simulink library "RobotStateLibrary_R2020b"  (R2020b)
settings: Solver=VariableStepAuto  StartTime=0.0  StopTime=10.0  RelTol=1e-3
undefined symbols (not defined in the file or in its folder): Aeq_add, baseFrameName1, basePosePortName, beq_add, config, Config, ConfigRobot1, configSafety, contactFrame1Name, contactFrame2Name, frame1, frame2, frame3, frame4, frameName2, gainStruct, RegStruct, regularization, sampleTime, tollerance, useConstraint, weight
libraries: WBToolboxLibrary x38, $bdroot x32
(part 1 of 2)
settings Model: Creator=lorenzorapetti  LastModifiedBy=lorenzorapetti

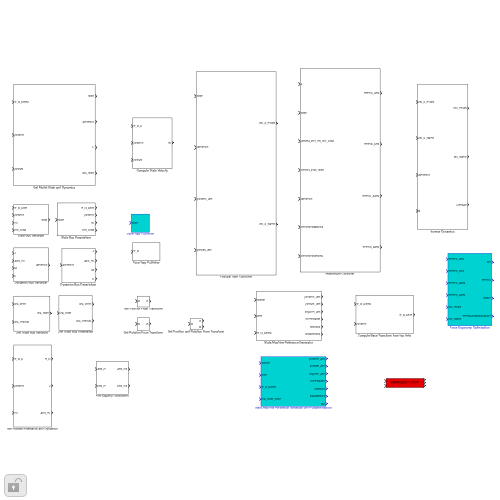
[thumbnail: Simulink's stored preview of the top-level diagram]
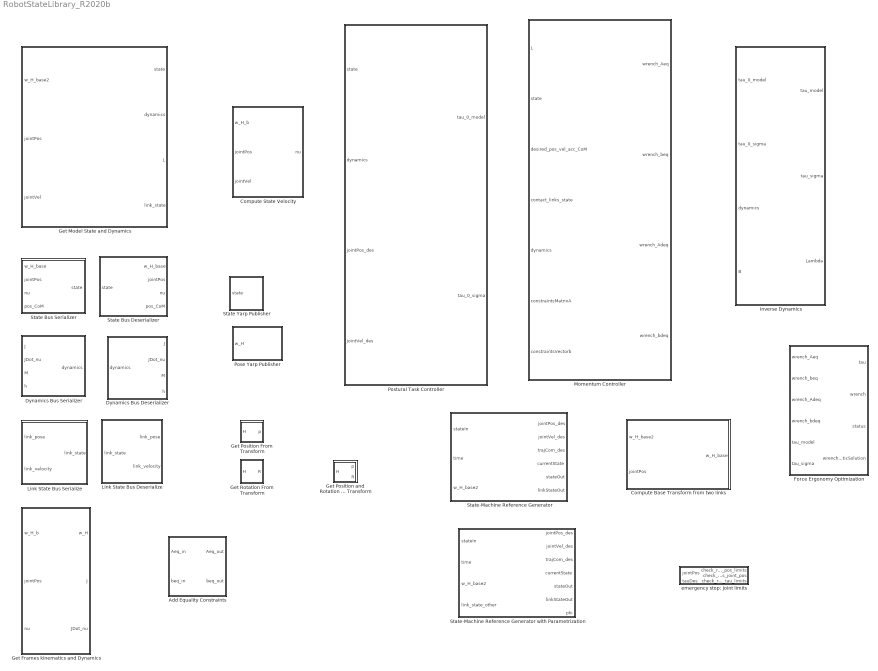
== system RobotStateLibrary_R2020b ==
  Add Equality Constraints : Subsystem  mask{Aeq_add=Aeq_add, beq_add=beq_add}
      mask prompts: Aeq_add "Additional Constraints A"; beq_add "Additional Constraints b"
  Compute Base Transform from two links : Subsystem  mask{frameName1=baseFrameName1, frameName2=frameName2}
      mask prompts: frameName1 "Frame name 1"; frameName2 "Frame name 2"
      mask TypeOptions frameName1: Relative transform base2_H_base/frameName
      mask TypeOptions frameName2: Relative transform base2_H_base1/frameName
  Compute State Velocity : Subsystem  mask{frameName1=contactFrame1Name, frameName2=contactFrame2Name, regularization=regularization}
      mask prompts: frameName1 "Contact Frame 1"; frameName2 "Contact Frame 2"
      mask TypeOptions frameName1: Contacts Jacobians/Jacobian Contact 1/frameName
      mask TypeOptions frameName2: Contacts Jacobians/Jacobian Contact 2/frameName
  Dynamics Bus Deserializer : Subsystem
  Dynamics Bus Serializer : Subsystem
  Force Ergonomy Optimization : Subsystem  mask{InvTol=tollerance, regularizationHessian=regularization, minimizationWeight=weight}
      mask prompts: InvTol "Pseudoinverse Tollerance"; regularizationHessian "Regularization Hessian"; minimizationWeight "Minimization Weight"
  Get Frames kinematics and Dynamics : Subsystem  mask{frame1=frame1, frame2=frame2, frame3=frame3, frame4=frame4, nDoF=1}
      mask prompts: frame1 "Frame 1"; frame2 "Frame 2"; frame3 "Frame 3"; frame4 "Frame 4"; nDoF "Model DoF"
      mask TypeOptions nDoF:
      | CoM6D ->
      | CoMXYZ3/OutputSizes
  Get Model State and Dynamics : Subsystem  mask{nDoF=1, regularization=0, contactFrame1Name=[], contactFrame2Name=[], frame1=[], frame2=[], frame3=[], frame4=[]}
      mask prompts: nDoF "Model DoF"; regularization "Base Velocity Regularization"; contactFrame1Name "Contact Frame 1"; contactFrame2Name "Contact Frame 2"; frame1 "Frame 1"; frame2 "Frame 2"; frame3 "Frame 3"; frame4 "Frame 4"
      mask TypeOptions nDoF: Get Frames kinematics and Dynamics/nDoF | Get Model Kinematics and Dynamics/nDoF
      mask TypeOptions regularization: Compute State Velocity/regularization
      mask TypeOptions contactFrame1Name: Compute State Velocity/frameName1
      mask TypeOptions contactFrame2Name: Compute State Velocity/frameName2
      mask TypeOptions frame1: Get Frames kinematics and Dynamics/frame1
      mask TypeOptions frame2: Get Frames kinematics and Dynamics/frame2
      mask TypeOptions frame3: Get Frames kinematics and Dynamics/frame3
      mask TypeOptions frame4: Get Frames kinematics and Dynamics/frame4
      mask DialogControl Container4 Prompt: Base Velocity Parameters
      mask DialogControl Container3 Prompt: Contact Frames
      mask DialogControl Container5 Prompt: Frames
  Get Position From Transform : Subsystem
  Get Position and Rotation From Transform : Subsystem
  Get Rotation From Transform : Subsystem
  Inverse Dynamics : Subsystem  mask{Reg=RegStruct, fixedLinkVelcityComponents=0}
      mask prompts: Reg "Regularization Values"; fixedLinkVelcityComponents "Fixed Link Velocity Components"
  Link State Bus Deserialize : Subsystem
  Link State Bus Serialize : Subsystem
  Momentum Controller : Subsystem  mask{GainMomentum=gainStruct, linksUseConstraintMatrix=useConstraint}
      mask prompts: GainMomentum "Momentum Control Gain"; linksUseConstraintMatrix "Use Force Constraint on Links"
  Pose Yarp Publisher : Subsystem  mask{portName=basePosePortName}
      mask prompts: portName "Pose Port Name"
      mask TypeOptions portName: base pose/portName
  Postural Task Controller : Subsystem  mask{GainPostural=gainStruct}
      mask prompts: GainPostural "Postural Task Gain"
  State Bus Deserializer : Subsystem
  State Bus Serializer : Subsystem
  State Yarp Publisher : Subsystem  mask{basePosePortName='/portname', jointPosPortName='/portname', nuPortName='/portname', posCoMPortName='/portname'}
      mask prompts: basePosePortName "Base Pose Port Name"; jointPosPortName "Joint Position Port Name"; nuPortName "State Velocity Port Name"; posCoMPortName "CoM Position Port Name"
      mask TypeOptions basePosePortName: Pose Yarp Publisher/portName
      mask TypeOptions jointPosPortName: joint position/portName
      mask TypeOptions nuPortName: nu/portName
      mask TypeOptions posCoMPortName: CoM position/portName
  State-Machine Reference Generator : Subsystem  mask{configStateMachine=config, sampleTime=sampleTime, frameName1=baseFrameName1, frameName2=baseFrameName1, regularization=regularization, nDoF=1, frame1=frame1, frame2=frame2, frame3=frame3, frame4=frame4}
      mask prompts: configStateMachine "State Machine Configuration"; sampleTime "Sample Time"; frameName1 "Contact Frame 1"; frameName2 "Contact Frame 2"; regularization "Base Veocity Regularization"; nDoF "Model DoF"; frame1 "Frame 1"; frame2 "Frame 2"; frame3 "Frame 3"; frame4 "Frame 4"
      mask TypeOptions sampleTime: MinimumJerkTrajectoryGenerator1/sampleTime | MinimumJerkTrajectoryGenerator2/sampleTime
      mask TypeOptions frameName1: Compute Base Transform from two links/frameName1 | Compute State Velocity/frameName1
      mask TypeOptions frameName2: Compute Base Transform from two links/frameName2 | Compute State Velocity/frameName2
      mask TypeOptions regularization: Compute State Velocity/regularization
      mask TypeOptions nDoF: Get Frames kinematics and Dynamics/nDoF
      mask TypeOptions frame1: Get Frames kinematics and Dynamics/frame1
      mask TypeOptions frame2: Get Frames kinematics and Dynamics/frame2
      mask TypeOptions frame3: Get Frames kinematics and Dynamics/frame3
      mask TypeOptions frame4: Get Frames kinematics and Dynamics/frame4
      mask DialogControl Container3 Prompt: Frames
  State-Machine Reference Generator with Parametrization : Subsystem  mask{configStateMachine=config, frameName1=frame1, frameName2=frame2, regularization=regularization, nDoF=ROBOT_DOF, frame1=frame1, frame2=frame2, frame3=frame3, frame4=frame4, settlingTime=1, sampleTime=1}
      mask prompts: configStateMachine "State Machine Configuration"; frameName1 "Contact Frame 1"; frameName2 "Contact Frame 2"; regularization "Base Veocity Regularization"; nDoF "Model DoF"; frame1 "Frame 1"; frame2 "Frame 2"; frame3 "Frame 3"; frame4 "Frame 4"; settlingTime "Settling Time"; sampleTime "Sample Time"
      mask TypeOptions frameName1: Compute Output State/frameName1 | Compute CoM Trajectory/frameName1
      mask TypeOptions frameName2: Compute Output State/frameName2 | Compute CoM Trajectory/frameName2
      mask TypeOptions regularization: Compute Output State/regularization
      mask TypeOptions nDoF: Compute Output State/nDoF
      mask TypeOptions frame1: Compute Output State/frame1
      mask TypeOptions frame2: Compute Output State/frame2
      mask TypeOptions frame3: Compute Output State/frame3
      mask TypeOptions frame4: Compute Output State/frame4
      mask TypeOptions settlingTime: Compute CoM Trajectory/settlingTime | Compute Output State/settlingTime
      mask TypeOptions sampleTime: Compute CoM Trajectory/sampleTime | Compute Output State/sampleTime
      mask DialogControl Container3 Prompt: Frames
      mask DialogControl Container4 Prompt: MinimumJerk
  emergency stop: joint limits : Subsystem  mask{Safety=configSafety}
      mask prompts: Safety "ConfigSafety"
      mask Display: disp('EMERGENCY STOP')

== system RobotStateLibrary_R2020b/Add Equality Constraints ==
  Aeq_in : Inport
  beq_in : Inport  Port=2
  Constant : Constant  Value=Aeq_add
  Constant1 : Constant  Value=beq_add
  Matrix Concatenate : Concatenate  Mode=Multidimensional array
  Matrix Concatenate1 : Concatenate  Mode=Multidimensional array
  Aeq_out : Outport
  beq_out : Outport  Port=2
  wires:
  Aeq_in/1 -> Matrix Concatenate/1
  Constant/1 -> Matrix Concatenate/2
  Matrix Concatenate/1 -> Aeq_out/1
  beq_in/1 -> Matrix Concatenate1/1
  Constant1/1 -> Matrix Concatenate1/2
  Matrix Concatenate1/1 -> beq_out/1

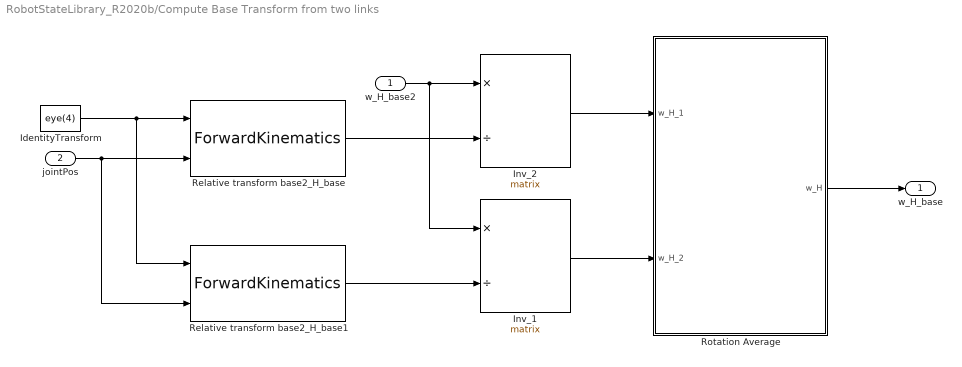
== system RobotStateLibrary_R2020b/Compute Base Transform from two links ==
  w_H_base2 : Inport
  jointPos : Inport  Port=2
  IdentityTransform : Constant  Value=eye(4)
  Inv_1 : Product  Inputs=*/  Multiplication=Matrix(*)
  Inv_2 : Product  Inputs=*/  Multiplication=Matrix(*)
  Relative transform base2_H_base : WBToolboxLibrary/Model/Kinematics/ForwardKinematics  frameName=frameName1
      settings: SourceProductName=WholeBodyToolbox
  Relative transform base2_H_base1 : WBToolboxLibrary/Model/Kinematics/ForwardKinematics  frameName=frameName2
      settings: SourceProductName=WholeBodyToolbox
  Rotation Average : MATLAB Function  TreatAsAtomicUnit=on
  w_H_base : Outport
  wires:
  w_H_base2/1 -> Inv_1/1, Inv_2/1
  jointPos/1 -> Relative transform base2_H_base1/2, Relative transform base2_H_base/2
  Relative transform base2_H_base/1 -> Inv_2/2
  IdentityTransform/1 -> Relative transform base2_H_base1/1, Relative transform base2_H_base/1
  Relative transform base2_H_base1/1 -> Inv_1/2
  Rotation Average/1(w_H) -> w_H_base/1
  Inv_2/1 -> Rotation Average/1(w_H_1)
  Inv_1/1 -> Rotation Average/2(w_H_2)

== system RobotStateLibrary_R2020b/Compute State Velocity ==
  w_H_b : Inport
  jointPos : Inport  Port=2
  jointVel : Inport  Port=3
  Compute Base Velocity : MATLAB Function  TreatAsAtomicUnit=on
  Contacts Jacobians : Subsystem
  Mux : Mux  Inputs=2
  nu : Outport  VectorParamsAs1DForOutWhenUnconnected=off
  wires:
  jointVel/1 -> Mux/2, Compute Base Velocity/3(jointVel)
  Mux/1 -> nu/1
  Compute Base Velocity/1(nu_b) -> Mux/1
  jointPos/1 -> Contacts Jacobians/1(jointPos)
  w_H_b/1 -> Contacts Jacobians/2(w_H_b)
  Contacts Jacobians/1(J_contact_1) -> Compute Base Velocity/1(J_contact_1)
  Contacts Jacobians/2(J_contact_2) -> Compute Base Velocity/2(J_contact_2)

== system RobotStateLibrary_R2020b/Dynamics Bus Deserializer ==
  dynamics : Inport
  Bus Selector : BusSelector  OutputSignals=J,JDot_nu,M,h
  J : Outport
  JDot_nu : Outport  Port=2
  M : Outport  Port=3
  h : Outport  Port=4
  wires:
  Bus Selector/1 -> J/1  "<J>"
  Bus Selector/4 -> h/1  "<h>"
  dynamics/1 -> Bus Selector/1
  Bus Selector/3 -> M/1  "<M>"
  Bus Selector/2 -> JDot_nu/1  "<JDot_nu>"

== system RobotStateLibrary_R2020b/Dynamics Bus Serializer ==
  J : Inport
  JDot_nu : Inport  Port=2
  M : Inport  Port=3
  h : Inport  Port=4
  Bus Creator : BusCreator  Inputs=4
  dynamics : Outport
  wires:
  JDot_nu/1 -> Bus Creator/2  "JDot_nu"
  h/1 -> Bus Creator/4  "h"
  J/1 -> Bus Creator/1  "J"
  Bus Creator/1 -> dynamics/1
  M/1 -> Bus Creator/3  "M"

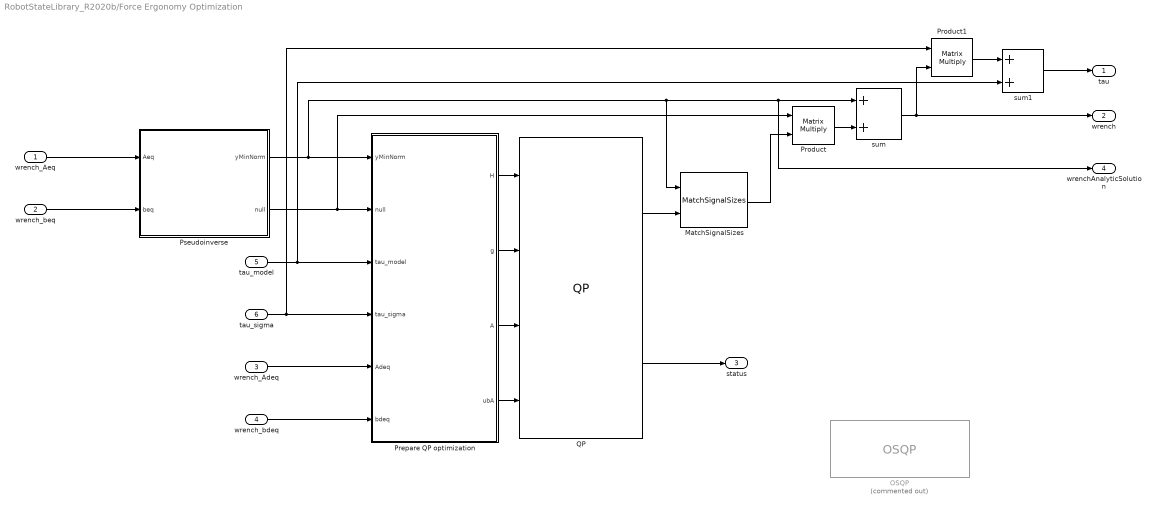
== system RobotStateLibrary_R2020b/Force Ergonomy Optimization ==
  wrench_Aeq : Inport
  wrench_beq : Inport  Port=2
  wrench_Adeq : Inport  Port=3
  wrench_bdeq : Inport  Port=4
  tau_model : Inport  Port=5
  tau_sigma : Inport  Port=6
  MatchSignalSizes : WBToolboxLibrary/Utilities/MatchSignalSizes
      settings: SourceProductName=WholeBodyToolbox
  OSQP : WBToolboxLibrary/Utilities/OSQP  Commented=on  lbA=off  ubA=on  lb=off  ub=off  computeObjVal=off  stopIfFails=off
      settings: SourceProductName=WholeBodyToolbox
  Prepare QP optimization : MATLAB Function  TreatAsAtomicUnit=on
  Product : Product  Multiplication=Matrix(*)
  Product1 : Product  Multiplication=Matrix(*)
  Pseudoinverse : MATLAB Function  TreatAsAtomicUnit=on
  QP : WBToolboxLibrary/Utilities/QP  lbA=off  ubA=on  lb=off  ub=off  computeObjVal=off  stopIfFails=off
      settings: SourceProductName=WholeBodyToolbox
  sum : Sum
  sum1 : Sum
  tau : Outport
  wrench : Outport  Port=2
  status : Outport  Port=3
  wrenchAnalyticSolution : Outport  Port=4
  wires:
  wrench_Aeq/1 -> Pseudoinverse/1(Aeq)
  wrench_beq/1 -> Pseudoinverse/2(beq)
  Pseudoinverse/1(yMinNorm) -> MatchSignalSizes/1, wrenchAnalyticSolution/1, sum/1, Prepare QP optimization/1(yMinNorm)
  sum1/1 -> tau/1
  Pseudoinverse/2(null) -> Product/1, Prepare QP optimization/2(null)
  wrench_Adeq/1 -> Prepare QP optimization/5(Adeq)
  wrench_bdeq/1 -> Prepare QP optimization/6(bdeq)
  tau_model/1 -> sum1/2, Prepare QP optimization/3(tau_model)
  tau_sigma/1 -> Product1/1, Prepare QP optimization/4(tau_sigma)
  Prepare QP optimization/4(ubA) -> QP/4
  Prepare QP optimization/3(A) -> QP/3
  Prepare QP optimization/2(g) -> QP/2
  Prepare QP optimization/1(H) -> QP/1
  Product/1 -> sum/2
  sum/1 -> wrench/1, Product1/2
  Product1/1 -> sum1/1
  MatchSignalSizes/1 -> Product/2
  QP/1 -> MatchSignalSizes/2
  QP/2 -> status/1

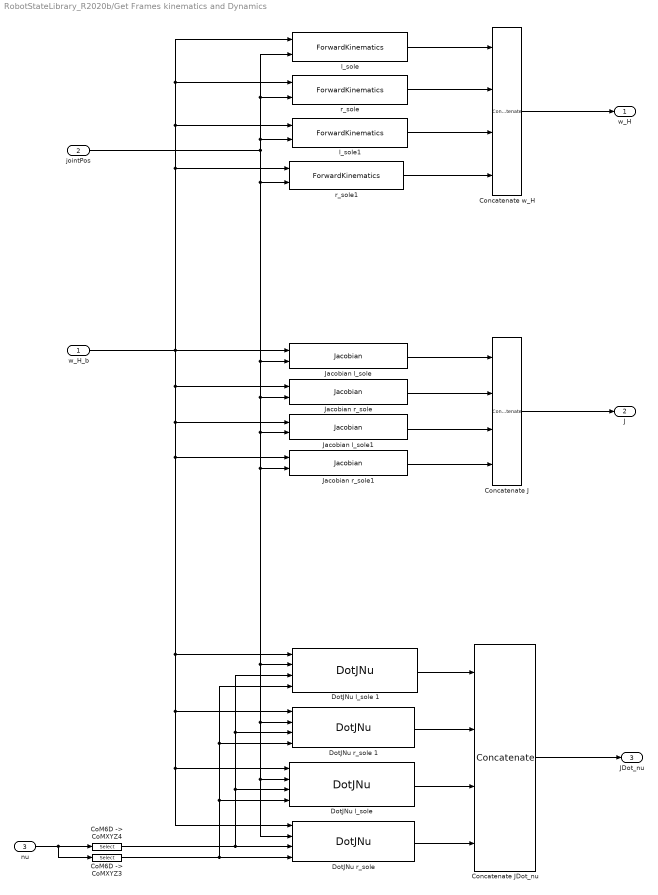
== system RobotStateLibrary_R2020b/Get Frames kinematics and Dynamics ==
  w_H_b : Inport
  jointPos : Inport  Port=2
  nu : Inport  Port=3
  "CoM6D -> CoMXYZ3" : Selector  IndexOptions=Starting index (dialog)  Indices=7  OutputSizes=1
  "CoM6D -> CoMXYZ4" : Selector  IndexOptions=Index vector (dialog)  Indices=[1 2 3 4 5 6]  OutputSizes=1
  Concatenate J : Concatenate  NumInputs=4  Mode=Multidimensional array
  Concatenate JDot_nu : Concatenate  NumInputs=4  Mode=Multidimensional array
  Concatenate w_H : Concatenate  NumInputs=4  Mode=Multidimensional array
  "DotJNu l_sole " : WBToolboxLibrary/Model/Jacobians/DotJNu  frameName=frame3
      settings: SourceProductName=WholeBodyToolbox
  DotJNu l_sole 1 : WBToolboxLibrary/Model/Jacobians/DotJNu  frameName=frame1
      settings: SourceProductName=WholeBodyToolbox
  "DotJNu r_sole " : WBToolboxLibrary/Model/Jacobians/DotJNu  frameName=frame4
      settings: SourceProductName=WholeBodyToolbox
  DotJNu r_sole 1 : WBToolboxLibrary/Model/Jacobians/DotJNu  frameName=frame2
      settings: SourceProductName=WholeBodyToolbox
  Jacobian l_sole : WBToolboxLibrary/Model/Jacobians/Jacobian  frameName=frame1
      settings: SourceProductName=WholeBodyToolbox
  Jacobian l_sole1 : WBToolboxLibrary/Model/Jacobians/Jacobian  frameName=frame3
      settings: SourceProductName=WholeBodyToolbox
  Jacobian r_sole : WBToolboxLibrary/Model/Jacobians/Jacobian  frameName=frame2
      settings: SourceProductName=WholeBodyToolbox
  Jacobian r_sole1 : WBToolboxLibrary/Model/Jacobians/Jacobian  frameName=frame4
      settings: SourceProductName=WholeBodyToolbox
  l_sole : WBToolboxLibrary/Model/Kinematics/ForwardKinematics  frameName=frame1
      settings: SourceProductName=WholeBodyToolbox
  l_sole1 : WBToolboxLibrary/Model/Kinematics/ForwardKinematics  frameName=frame3
      settings: SourceProductName=WholeBodyToolbox
  r_sole : WBToolboxLibrary/Model/Kinematics/ForwardKinematics  frameName=frame2
      settings: SourceProductName=WholeBodyToolbox
  r_sole1 : WBToolboxLibrary/Model/Kinematics/ForwardKinematics  frameName=frame4
      settings: SourceProductName=WholeBodyToolbox
  w_H : Outport  VectorParamsAs1DForOutWhenUnconnected=off
  J : Outport  Port=2  VectorParamsAs1DForOutWhenUnconnected=off
  JDot_nu : Outport  Port=3  VectorParamsAs1DForOutWhenUnconnected=off
  wires:
  "CoM6D -> CoMXYZ3"/1 -> "DotJNu l_sole "/4, DotJNu r_sole 1/4, DotJNu l_sole 1/4, "DotJNu r_sole "/4
  "CoM6D -> CoMXYZ4"/1 -> "DotJNu l_sole "/3, DotJNu r_sole 1/3, DotJNu l_sole 1/3, "DotJNu r_sole "/3
  nu/1 -> "CoM6D -> CoMXYZ3"/1, "CoM6D -> CoMXYZ4"/1
  Jacobian l_sole/1 -> Concatenate J/1
  Jacobian r_sole/1 -> Concatenate J/2
  "DotJNu l_sole "/1 -> Concatenate JDot_nu/3
  "DotJNu r_sole "/1 -> Concatenate JDot_nu/4
  Jacobian l_sole1/1 -> Concatenate J/3
  Jacobian r_sole1/1 -> Concatenate J/4
  DotJNu r_sole 1/1 -> Concatenate JDot_nu/2
  DotJNu l_sole 1/1 -> Concatenate JDot_nu/1
  w_H_b/1 -> Jacobian l_sole/1, r_sole1/1, l_sole1/1, r_sole/1, l_sole/1, DotJNu l_sole 1/1, DotJNu r_sole 1/1, "DotJNu r_sole "/1, "DotJNu l_sole "/1, Jacobian r_sole1/1, Jacobian l_sole1/1, Jacobian r_sole/1
  jointPos/1 -> DotJNu l_sole 1/2, DotJNu r_sole 1/2, "DotJNu r_sole "/2, "DotJNu l_sole "/2, Jacobian r_sole1/2, Jacobian l_sole1/2, Jacobian r_sole/2, Jacobian l_sole/2, r_sole1/2, r_sole/2, l_sole/2, l_sole1/2
  Concatenate w_H/1 -> w_H/1
  l_sole/1 -> Concatenate w_H/1
  r_sole/1 -> Concatenate w_H/2
  l_sole1/1 -> Concatenate w_H/3
  r_sole1/1 -> Concatenate w_H/4
  Concatenate J/1 -> J/1
  Concatenate JDot_nu/1 -> JDot_nu/1

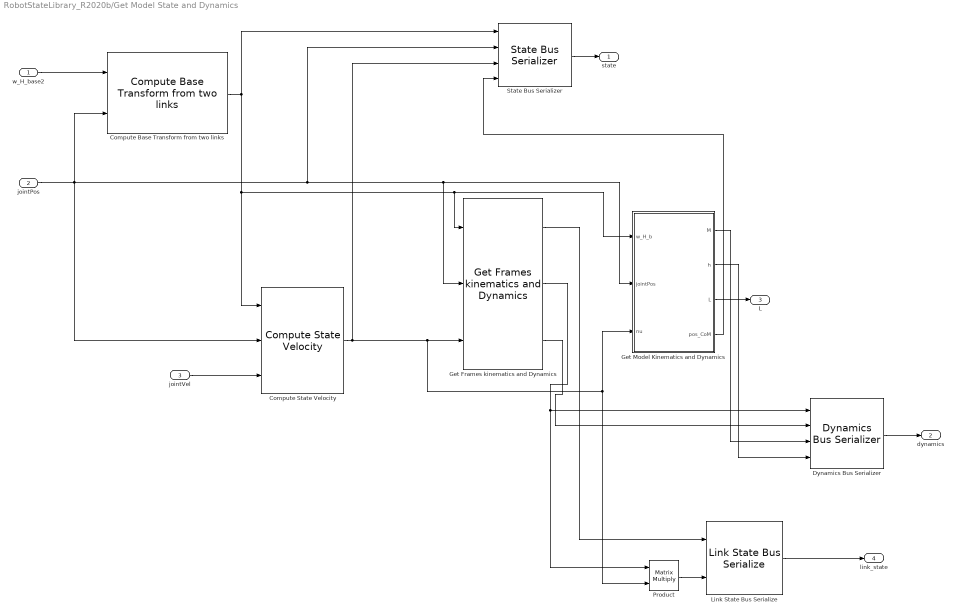
== system RobotStateLibrary_R2020b/Get Model State and Dynamics ==
  w_H_base2 : Inport
  jointPos : Inport  Port=2
  jointVel : Inport  Port=3
  Compute Base Transform from two links : $bdroot/Compute Base Transform from two links  frameName1=contactFrame1Name  frameName2=contactFrame2Name
  Compute State Velocity : $bdroot/Compute State Velocity  frameName1=contactFrame1Name  frameName2=contactFrame2Name  regularization=regularization
  Dynamics Bus Serializer : $bdroot/Dynamics Bus Serializer  SystemSampleTime=-1  VariantActivationTime=update diagram  Latency=0  AutoFrameSizeCalculation=off
  Get Frames kinematics and Dynamics : $bdroot/Get Frames kinematics and Dynamics  frame1=frame1  frame2=frame2  frame3=frame3  frame4=frame4  nDoF=1
  Get Model Kinematics and Dynamics : Subsystem  mask{nDoF=1}
      mask prompts: nDoF "Model DoF"
      mask TypeOptions nDoF:
      | CoM6D ->
      | CoMXYZ1/OutputSizes
  Link State Bus Serialize : $bdroot/Link State Bus Serialize  SystemSampleTime=-1  VariantActivationTime=update diagram  Latency=0  AutoFrameSizeCalculation=off
  Product : Product  Multiplication=Matrix(*)
  State Bus Serializer : $bdroot/State Bus Serializer  SystemSampleTime=-1  VariantActivationTime=update diagram  Latency=0  AutoFrameSizeCalculation=off
  state : Outport
  dynamics : Outport  Port=2
  L : Outport  Port=3
  link_state : Outport  Port=4
  wires:
  Compute State Velocity/1 -> State Bus Serializer/3, Get Frames kinematics and Dynamics/3, Get Model Kinematics and Dynamics/3(nu), Product/2
  Get Model Kinematics and Dynamics/1(M) -> Dynamics Bus Serializer/3
  Get Model Kinematics and Dynamics/3(L) -> L/1
  Get Model Kinematics and Dynamics/4(pos_CoM) -> State Bus Serializer/4
  Get Frames kinematics and Dynamics/1 -> Link State Bus Serialize/1
  Get Frames kinematics and Dynamics/3 -> Dynamics Bus Serializer/2
  Compute Base Transform from two links/1 -> State Bus Serializer/1, Compute State Velocity/1, Get Frames kinematics and Dynamics/1, Get Model Kinematics and Dynamics/1(w_H_b)
  jointPos/1 -> Compute State Velocity/2, Compute Base Transform from two links/2, State Bus Serializer/2, Get Frames kinematics and Dynamics/2, Get Model Kinematics and Dynamics/2(jointPos)
  Get Frames kinematics and Dynamics/2 -> Product/1, Dynamics Bus Serializer/1
  Get Model Kinematics and Dynamics/2(h) -> Dynamics Bus Serializer/4
  w_H_base2/1 -> Compute Base Transform from two links/1
  jointVel/1 -> Compute State Velocity/3
  State Bus Serializer/1 -> state/1
  Dynamics Bus Serializer/1 -> dynamics/1
  Link State Bus Serialize/1 -> link_state/1
  Product/1 -> Link State Bus Serialize/2

== system RobotStateLibrary_R2020b/Get Position From Transform ==
  H : Inport
  GetPosition : Selector  NumberOfDimensions=2  InputPortWidth=3  IndexOptions=Index vector (dialog),Index vector (dialog)  Indices=[1 2 3],4  OutputSizes=1,1
  p : Outport
  wires:
  GetPosition/1 -> p/1
  H/1 -> GetPosition/1

== system RobotStateLibrary_R2020b/Get Position and Rotation From Transform ==
  H : Inport
  Get Position From Transform : $bdroot/Get Position From Transform  SystemSampleTime=-1  VariantActivationTime=update diagram  Latency=0  AutoFrameSizeCalculation=off
  Get Rotation From Transform : $bdroot/Get Rotation From Transform  SystemSampleTime=-1  VariantActivationTime=update diagram  Latency=0  AutoFrameSizeCalculation=off
  p : Outport
  R : Outport  Port=2
  wires:
  Get Position From Transform/1 -> p/1
  Get Rotation From Transform/1 -> R/1
  H/1 -> Get Position From Transform/1, Get Rotation From Transform/1

== system RobotStateLibrary_R2020b/Get Rotation From Transform ==
  H : Inport
  GetPosition : Selector  NumberOfDimensions=2  InputPortWidth=3  IndexOptions=Index vector (dialog),Index vector (dialog)  Indices=[1 2 3],4  OutputSizes=1,1
  R : Outport
  wires:
  GetPosition/1 -> R/1
  H/1 -> GetPosition/1

== system RobotStateLibrary_R2020b/Inverse Dynamics ==
  tau_0_model : Inport
  tau_0_sigma : Inport  Port=2
  dynamics : Inport  Port=3
  B : Inport  Port=4
  Dynamics Bus Deserializer : $bdroot/Dynamics Bus Deserializer  SystemSampleTime=-1  VariantActivationTime=update diagram  Latency=0  AutoFrameSizeCalculation=off
  Inverse Dynamics : MATLAB Function  TreatAsAtomicUnit=on
  tau_model : Outport
  tau_sigma : Outport  Port=2
  Lambda : Outport  Port=3
  wires:
  dynamics/1 -> Dynamics Bus Deserializer/1
  Inverse Dynamics/1(tau_model) -> tau_model/1
  Inverse Dynamics/2(tau_sigma) -> tau_sigma/1
  Dynamics Bus Deserializer/1 -> Inverse Dynamics/3(J)
  Dynamics Bus Deserializer/2 -> Inverse Dynamics/4(JDot_nu)
  Dynamics Bus Deserializer/3 -> Inverse Dynamics/5(M)
  Dynamics Bus Deserializer/4 -> Inverse Dynamics/6(h)
  tau_0_sigma/1 -> Inverse Dynamics/2(tau_0_sigma)
  tau_0_model/1 -> Inverse Dynamics/1(tau_0_model)
  B/1 -> Inverse Dynamics/7(B)
  Inverse Dynamics/3(Lambda) -> Lambda/1

== system RobotStateLibrary_R2020b/Link State Bus Deserialize ==
  link_state : Inport
  Bus Selector : BusSelector  OutputSignals=link_pose,link_velocity
  link_pose : Outport
  link_velocity : Outport  Port=2
  wires:
  Bus Selector/2 -> link_velocity/1  "<link_velocity>"
  link_state/1 -> Bus Selector/1
  Bus Selector/1 -> link_pose/1  "<link_pose>"

== system RobotStateLibrary_R2020b/Link State Bus Serialize ==
  link_pose : Inport
  link_velocity : Inport  Port=2
  Bus Creator : BusCreator  Inputs=2
  link_state : Outport
  wires:
  Bus Creator/1 -> link_state/1  "link_state"
  link_velocity/1 -> Bus Creator/2  "link_velocity"
  link_pose/1 -> Bus Creator/1  "link_pose"

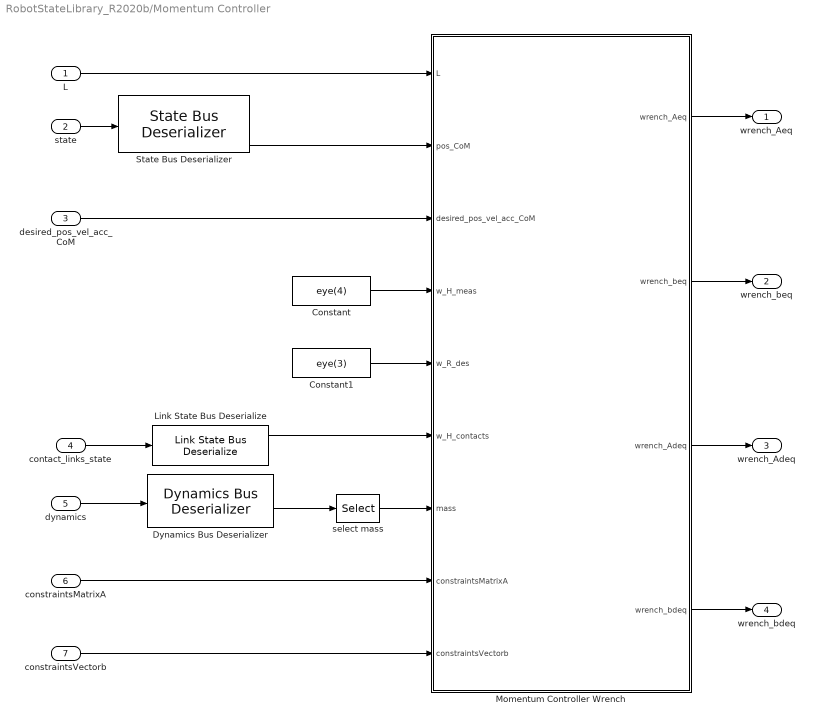
== system RobotStateLibrary_R2020b/Momentum Controller ==
  L : Inport
  state : Inport  Port=2
  desired_pos_vel_acc_CoM : Inport  Port=3
  contact_links_state : Inport  Port=4
  dynamics : Inport  Port=5
  constraintsMatrixA : Inport  Port=6
  constraintsVectorb : Inport  Port=7
  Constant : Constant  Value=eye(4)
  Constant1 : Constant  Value=eye(3)
  Dynamics Bus Deserializer : $bdroot/Dynamics Bus Deserializer  SystemSampleTime=-1  VariantActivationTime=update diagram  Latency=0  AutoFrameSizeCalculation=off
  Link State Bus Deserialize : $bdroot/Link State Bus Deserialize  SystemSampleTime=-1  VariantActivationTime=update diagram  Latency=0  AutoFrameSizeCalculation=off
  Momentum Controller Wrench : MATLAB Function  TreatAsAtomicUnit=on
  State Bus Deserializer : $bdroot/State Bus Deserializer  SystemSampleTime=-1  VariantActivationTime=update diagram  Latency=0  AutoFrameSizeCalculation=off
  select mass : Selector  NumberOfDimensions=2  InputPortWidth=3  IndexOptions=Index vector (dialog),Index vector (dialog)  Indices=1,1  OutputSizes=1,1
  wrench_Aeq : Outport
  wrench_beq : Outport  Port=2
  wrench_Adeq : Outport  Port=3
  wrench_bdeq : Outport  Port=4
  wires:
  Momentum Controller Wrench/2(wrench_beq) -> wrench_beq/1
  Momentum Controller Wrench/1(wrench_Aeq) -> wrench_Aeq/1
  Momentum Controller Wrench/3(wrench_Adeq) -> wrench_Adeq/1
  Momentum Controller Wrench/4(wrench_bdeq) -> wrench_bdeq/1
  L/1 -> Momentum Controller Wrench/1(L)
  desired_pos_vel_acc_CoM/1 -> Momentum Controller Wrench/3(desired_pos_vel_acc_CoM)
  constraintsMatrixA/1 -> Momentum Controller Wrench/8(constraintsMatrixA)
  constraintsVectorb/1 -> Momentum Controller Wrench/9(constraintsVectorb)
  state/1 -> State Bus Deserializer/1
  State Bus Deserializer/4 -> Momentum Controller Wrench/2(pos_CoM)
  contact_links_state/1 -> Link State Bus Deserialize/1
  Link State Bus Deserialize/1 -> Momentum Controller Wrench/6(w_H_contacts)
  select mass/1 -> Momentum Controller Wrench/7(mass)
  dynamics/1 -> Dynamics Bus Deserializer/1
  Dynamics Bus Deserializer/3 -> select mass/1
  Constant/1 -> Momentum Controller Wrench/4(w_H_meas)
  Constant1/1 -> Momentum Controller Wrench/5(w_R_des)

== system RobotStateLibrary_R2020b/Pose Yarp Publisher ==
  w_H : Inport
  Transform Matrix to quaternion and position : MATLAB Function  TreatAsAtomicUnit=on
  base pose : WBToolboxLibrary/Utilities/YarpWrite  portName=portName  autoconnect=off  errorOnConnection=on
      settings: SourceProductName=WholeBodyToolbox
  wires:
  Transform Matrix to quaternion and position/1(q) -> base pose/1
  w_H/1 -> Transform Matrix to quaternion and position/1(w_H)

== system RobotStateLibrary_R2020b/Postural Task Controller ==
  state : Inport
  dynamics : Inport  Port=2
  jointPos_des : Inport  Port=3
  jointVel_des : Inport  Port=4
  Dynamics Bus Deserializer : $bdroot/Dynamics Bus Deserializer  SystemSampleTime=-1  VariantActivationTime=update diagram  Latency=0  AutoFrameSizeCalculation=off
  Postural Task Controller : MATLAB Function  TreatAsAtomicUnit=on
  State Bus Deserializer : $bdroot/State Bus Deserializer  SystemSampleTime=-1  VariantActivationTime=update diagram  Latency=0  AutoFrameSizeCalculation=off
  tau_0_model : Outport
  tau_0_sigma : Outport  Port=2
  wires:
  Dynamics Bus Deserializer/3 -> Postural Task Controller/4(M)
  Dynamics Bus Deserializer/1 -> Postural Task Controller/3(J)
  State Bus Deserializer/3 -> Postural Task Controller/2(nu)
  Dynamics Bus Deserializer/4 -> Postural Task Controller/5(h)
  Postural Task Controller/2(tau_0_sigma) -> tau_0_sigma/1
  jointPos_des/1 -> Postural Task Controller/6(jointPos_des)
  Postural Task Controller/1(tau_0_model) -> tau_0_model/1
  jointVel_des/1 -> Postural Task Controller/7(jointVel_des)
  State Bus Deserializer/2 -> Postural Task Controller/1(jointPos)
  state/1 -> State Bus Deserializer/1
  dynamics/1 -> Dynamics Bus Deserializer/1

== system RobotStateLibrary_R2020b/State Bus Deserializer ==
  state : Inport
  Bus Selector : BusSelector  OutputSignals=w_H_base,jointPos,nu,pos_CoM
  w_H_base : Outport
  jointPos : Outport  Port=2
  nu : Outport  Port=3
  pos_CoM : Outport  Port=4
  wires:
  Bus Selector/4 -> pos_CoM/1  "<pos_CoM>"
  Bus Selector/1 -> w_H_base/1  "<w_H_base>"
  Bus Selector/2 -> jointPos/1  "<jointPos>"
  Bus Selector/3 -> nu/1  "<nu>"
  state/1 -> Bus Selector/1

== system RobotStateLibrary_R2020b/State Bus Serializer ==
  w_H_base : Inport
  jointPos : Inport  Port=2
  nu : Inport  Port=3
  pos_CoM : Inport  Port=4
  Bus Creator : BusCreator  Inputs=4
  state : Outport
  wires:
  nu/1 -> Bus Creator/3  "nu"
  jointPos/1 -> Bus Creator/2  "jointPos"
  Bus Creator/1 -> state/1
  pos_CoM/1 -> Bus Creator/4  "pos_CoM"
  w_H_base/1 -> Bus Creator/1  "w_H_base"

== system RobotStateLibrary_R2020b/State Yarp Publisher ==
  state : Inport
  CoM position : WBToolboxLibrary/Utilities/YarpWrite  portName=posCoMPortName  autoconnect=off  errorOnConnection=on
      settings: SourceProductName=WholeBodyToolbox
  Pose Yarp Publisher : $bdroot/Pose Yarp Publisher  portName=basePosePortName
  State Bus Deserializer : $bdroot/State Bus Deserializer  SystemSampleTime=-1  VariantActivationTime=update diagram  Latency=0  AutoFrameSizeCalculation=off
  joint position : WBToolboxLibrary/Utilities/YarpWrite  portName=jointPosPortName  autoconnect=off  errorOnConnection=on
      settings: SourceProductName=WholeBodyToolbox
  nu : WBToolboxLibrary/Utilities/YarpWrite  portName=nuPortName  autoconnect=off  errorOnConnection=on
      settings: SourceProductName=WholeBodyToolbox
  wires:
  state/1 -> State Bus Deserializer/1
  State Bus Deserializer/1 -> Pose Yarp Publisher/1
  State Bus Deserializer/2 -> joint position/1
  State Bus Deserializer/3 -> nu/1
  State Bus Deserializer/4 -> CoM position/1

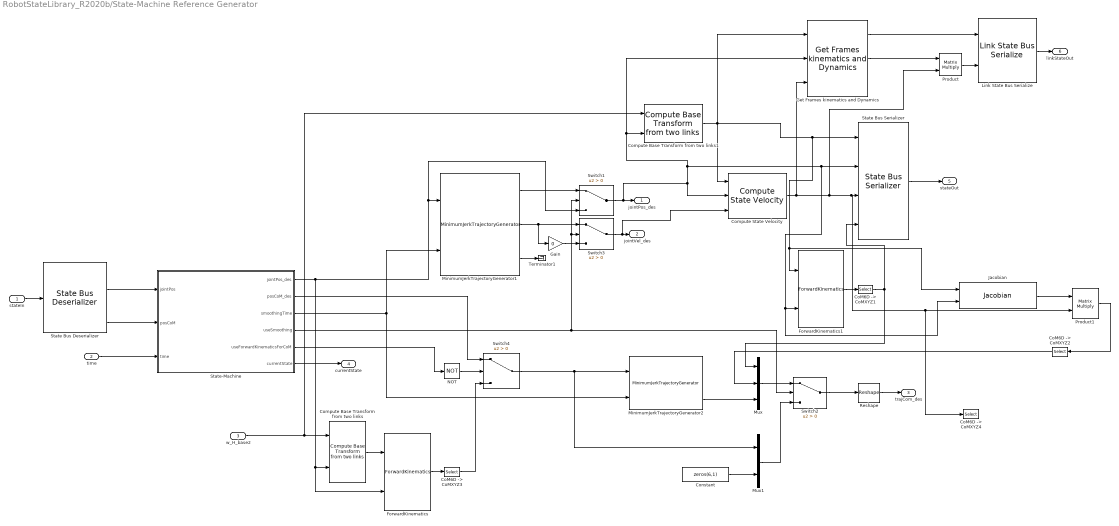
== system RobotStateLibrary_R2020b/State-Machine Reference Generator ==
  stateIn : Inport
  time : Inport  Port=2
  w_H_base2 : Inport  Port=3
  "CoM6D -> CoMXYZ1" : Selector  NumberOfDimensions=2  InputPortWidth=7  IndexOptions=Index vector (dialog),Index vector (dialog)  Indices=[1 2 3],[4]  OutputSizes=1,1
  "CoM6D -> CoMXYZ2" : Selector  InputPortWidth=7  IndexOptions=Index vector (dialog)  Indices=[1 2 3]  OutputSizes=1
  "CoM6D -> CoMXYZ3" : Selector  NumberOfDimensions=2  InputPortWidth=7  IndexOptions=Index vector (dialog),Index vector (dialog)  Indices=[1 2 3],[4]  OutputSizes=1,1
  "CoM6D -> CoMXYZ4" : Selector  IndexOptions=Index vector (dialog)  Indices=[1 2 3 4 5 6]  OutputSizes=1
  Compute Base Transform from two links : $bdroot/Compute Base Transform from two links  frameName1=frameName1  frameName2=frameName2
  Compute Base Transform from two links1 : $bdroot/Compute Base Transform from two links  frameName1=frameName1  frameName2=frameName2
  Compute State Velocity : $bdroot/Compute State Velocity  frameName1=frameName1  frameName2=frameName2  regularization=regularization
  Constant : Constant  Value=zeros(6,1)
  ForwardKinematics : WBToolboxLibrary/Model/Kinematics/ForwardKinematics  frameName='com'
      settings: SourceProductName=WholeBodyToolbox
  ForwardKinematics1 : WBToolboxLibrary/Model/Kinematics/ForwardKinematics  frameName='com'
      settings: SourceProductName=WholeBodyToolbox
  Gain : Gain  Gain=0
  Get Frames kinematics and Dynamics : $bdroot/Get Frames kinematics and Dynamics  frame1=frame1  frame2=frame2  frame3=frame3  frame4=frame4  nDoF=1
  Jacobian : WBToolboxLibrary/Model/Jacobians/Jacobian  frameName='com'
      settings: SourceProductName=WholeBodyToolbox
  Link State Bus Serialize : $bdroot/Link State Bus Serialize  SystemSampleTime=-1  VariantActivationTime=update diagram  Latency=0  AutoFrameSizeCalculation=off
  MinimumJerkTrajectoryGenerator1 : WBToolboxLibrary/Utilities/MinimumJerkTrajectoryGenerator  externalSettlingTime=on  settlingTime=0.01  sampleTime=sampleTime  resetOnSettlingTime=off  firstDerivatives=on  secondDerivatives=on  explicitInitialValue=off
      settings: SourceProductName=WholeBodyToolbox
  MinimumJerkTrajectoryGenerator2 : WBToolboxLibrary/Utilities/MinimumJerkTrajectoryGenerator  externalSettlingTime=on  settlingTime=0.01  sampleTime=sampleTime  resetOnSettlingTime=off  firstDerivatives=on  secondDerivatives=on  explicitInitialValue=off
      settings: SourceProductName=WholeBodyToolbox
  Mux : Mux  Inputs=3
  Mux1 : Mux  Inputs=2
  NOT : Logic  Operator=NOT  IconShape=distinctive  AllPortsSameDT=off  OutDataTypeStr=boolean
  Product : Product  Multiplication=Matrix(*)
  Product1 : Product  Multiplication=Matrix(*)
  Reshape : Reshape  OutputDimensionality=Customize  OutputDimensions=[3,3]
  State Bus Deserializer : $bdroot/State Bus Deserializer  SystemSampleTime=-1  VariantActivationTime=update diagram  Latency=0  AutoFrameSizeCalculation=off
  State Bus Serializer : $bdroot/State Bus Serializer  SystemSampleTime=-1  VariantActivationTime=update diagram  Latency=0  AutoFrameSizeCalculation=off
  State-Machine : MATLAB Function  TreatAsAtomicUnit=on
  Switch{1..4} (4 alike) : Switch  Criteria=u2 > Threshold
  Terminator1 : Terminator
  jointPos_des : Outport
  jointVel_des : Outport  Port=2
  trajCom_des : Outport  Port=3
  currentState : Outport  Port=4
  stateOut : Outport  Port=5
  linkStateOut : Outport  Port=6
  wires:
  time/1 -> State-Machine/3(time)
  State Bus Deserializer/2 -> State-Machine/1(jointPos)
  State Bus Deserializer/4 -> State-Machine/2(posCoM)
  stateIn/1 -> State Bus Deserializer/1
  MinimumJerkTrajectoryGenerator1/3 -> Terminator1/1
  State-Machine/1(jointPos_des) -> ForwardKinematics/2, Compute Base Transform from two links/2, Switch1/3, MinimumJerkTrajectoryGenerator1/1
  State-Machine/3(smoothingTime) -> MinimumJerkTrajectoryGenerator2/2, MinimumJerkTrajectoryGenerator1/2
  MinimumJerkTrajectoryGenerator2/3 -> Mux/3
  Reshape/1 -> trajCom_des/1
  State-Machine/4(useSmoothing) -> Switch2/2, Switch1/2, Switch3/2
  MinimumJerkTrajectoryGenerator1/2 -> Gain/1, Switch3/1
  MinimumJerkTrajectoryGenerator1/1 -> Switch1/1
  Gain/1 -> Switch3/3
  Switch2/1 -> Reshape/1
  Mux/1 -> Switch2/1
  Constant/1 -> Mux1/2
  Mux1/1 -> Switch2/3
  State-Machine/6(currentState) -> currentState/1
  w_H_base2/1 -> Compute Base Transform from two links1/1, Compute Base Transform from two links/1
  Compute Base Transform from two links/1 -> ForwardKinematics/1
  ForwardKinematics/1 -> "CoM6D -> CoMXYZ3"/1
  State-Machine/5(useForwardKinematicsForCoM) -> NOT/1
  Switch4/1 -> Mux1/1, MinimumJerkTrajectoryGenerator2/1
  NOT/1 -> Switch4/2
  State-Machine/2(posCoM_des) -> Switch4/1
  "CoM6D -> CoMXYZ3"/1 -> Switch4/3
  State Bus Serializer/1 -> stateOut/1
  Compute State Velocity/1 -> Get Frames kinematics and Dynamics/3, Product/2, "CoM6D -> CoMXYZ4"/1, Product1/2, State Bus Serializer/3
  Switch1/1 -> Compute State Velocity/2, Get Frames kinematics and Dynamics/2, Compute Base Transform from two links1/2, Jacobian/2, ForwardKinematics1/2, State Bus Serializer/2, jointPos_des/1
  Compute Base Transform from two links1/1 -> Compute State Velocity/1, Get Frames kinematics and Dynamics/1, Jacobian/1, ForwardKinematics1/1, State Bus Serializer/1
  Product/1 -> Link State Bus Serialize/2
  Get Frames kinematics and Dynamics/2 -> Product/1
  Link State Bus Serialize/1 -> linkStateOut/1
  Get Frames kinematics and Dynamics/1 -> Link State Bus Serialize/1
  ForwardKinematics1/1 -> "CoM6D -> CoMXYZ1"/1
  "CoM6D -> CoMXYZ1"/1 -> State Bus Serializer/4, Mux/1
  Jacobian/1 -> Product1/1
  Product1/1 -> "CoM6D -> CoMXYZ2"/1
  "CoM6D -> CoMXYZ2"/1 -> Mux/2
  Switch3/1 -> Compute State Velocity/3, jointVel_des/1

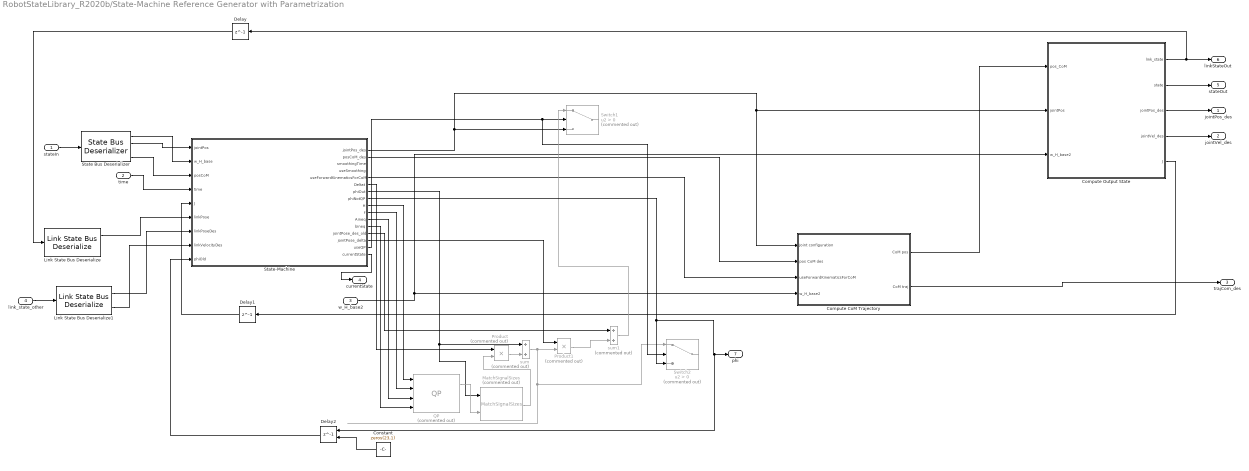
== system RobotStateLibrary_R2020b/State-Machine Reference Generator with Parametrization ==
  stateIn : Inport
  time : Inport  Port=2
  w_H_base2 : Inport  Port=3
  link_state_other : Inport  Port=4
  Compute CoM Trajectory : Subsystem  mask{frameName1=frameName1, frameName2=frameName2, settlingTime=settlingTime, sampleTime=sampleTime}
      mask prompts: frameName1 "Frame name 1"; frameName2 "Frame name 2"; settlingTime "Settling Time"; sampleTime "Sample Time"
      mask TypeOptions frameName1: Compute Base Transform from two links/frameName1
      mask TypeOptions frameName2: Compute Base Transform from two links/frameName2
      mask TypeOptions settlingTime: MinimumJerkTrajectoryGenerator/settlingTime
      mask TypeOptions sampleTime: MinimumJerkTrajectoryGenerator/sampleTime
      mask DialogControl MinimumJerkTraj Prompt: MinimumJerk
  Compute Output State : Subsystem  mask{frameName1=frameName1, frameName2=frameName2, nDoF=ROBOT_DOF, regularization=regularization, frame1=frame1, frame2=frame2, frame3=frame3, frame4=frame4, settlingTime=settlingTime, sampleTime=sampleTime}
      mask prompts: frameName1 "Contact Frame 1"; frameName2 "Contact Frame 2"; nDoF "Model DoF"; frame1 "Frame 1"; frame2 "Frame 2"; frame3 "Frame 3"; frame4 "Frame 4"; settlingTime "Settling Time"; sampleTime "Sample Time"
      mask TypeOptions frameName1: Compute Base Transform from two links1/frameName1 | Compute State Velocity/frameName1
      mask TypeOptions frameName2: Compute Base Transform from two links1/frameName2 | Compute State Velocity/frameName2
      mask TypeOptions nDoF: Get Frames kinematics and Dynamics/nDoF
      mask TypeOptions regularization: Compute State Velocity/regularization
      mask TypeOptions frame1: Get Frames kinematics and Dynamics/frame1
      mask TypeOptions frame2: Get Frames kinematics and Dynamics/frame2
      mask TypeOptions frame3: Get Frames kinematics and Dynamics/frame3
      mask TypeOptions frame4: Get Frames kinematics and Dynamics/frame4
      mask TypeOptions settlingTime: MinimumJerkTrajectoryGenerator/settlingTime
      mask TypeOptions sampleTime: MinimumJerkTrajectoryGenerator/sampleTime
      mask DialogControl Container3 Prompt: Frames
      mask DialogControl Container4 Prompt: MinJerk
  Constant : Constant  Value=zeros(23,1)
  Delay : Delay  DelayLength=1
  Delay1 : Delay  DelayLength=1
  Delay2 : Delay  DelayLength=1  InitialConditionSource=Input port
      settings: InputPortMap=u0,p4
  Link State Bus Deserialize : $bdroot/Link State Bus Deserialize  SystemSampleTime=-1  VariantActivationTime=update diagram  Latency=0  AutoFrameSizeCalculation=off
  Link State Bus Deserialize1 : $bdroot/Link State Bus Deserialize  SystemSampleTime=-1  VariantActivationTime=update diagram  Latency=0  AutoFrameSizeCalculation=off
  MatchSignalSizes : WBToolboxLibrary/Utilities/MatchSignalSizes  Commented=on
      settings: SourceProductName=WholeBodyToolbox
  Product : Product  Commented=on
  Product1 : Product  Commented=on
  QP : WBToolboxLibrary/Utilities/QP  Commented=on  lbA=off  ubA=on  lb=off  ub=off  computeObjVal=off  stopIfFails=off
      settings: SourceProductName=WholeBodyToolbox
  State Bus Deserializer : $bdroot/State Bus Deserializer  SystemSampleTime=-1  VariantActivationTime=update diagram  Latency=0  AutoFrameSizeCalculation=off
  State-Machine : MATLAB Function  TreatAsAtomicUnit=on
  Switch1 : Switch  Commented=on  Criteria=u2 > Threshold
  Switch2 : Switch  Commented=on  Criteria=u2 > Threshold
  sum : Sum  Commented=on
  sum1 : Sum  Commented=on
  jointPos_des : Outport
  jointVel_des : Outport  Port=2
  trajCom_des : Outport  Port=3
  currentState : Outport  Port=4
  stateOut : Outport  Port=5
  linkStateOut : Outport  Port=6
  phi : Outport  Port=7
  wires:
  w_H_base2/1 -> Compute Output State/3(w_H_base2), Compute CoM Trajectory/4(w_H_base2)
  State-Machine/16(currentState) -> currentState/1
  stateIn/1 -> State Bus Deserializer/1
  State Bus Deserializer/4 -> State-Machine/3(posCoM)
  State Bus Deserializer/2 -> State-Machine/1(jointPos)
  time/1 -> State-Machine/4(time)
  Compute Output State/1(link_state) -> Delay/1, linkStateOut/1
  Compute Output State/2(state) -> stateOut/1
  Compute Output State/3(jointPos_des) -> jointPos_des/1
  Compute Output State/4(jointVel_des) -> jointVel_des/1
  State-Machine/2(posCoM_des) -> Compute CoM Trajectory/2(pos CoM des)
  State-Machine/5(useForwardKinematicsForCoM) -> Compute CoM Trajectory/3(useForwardKinematicsForCoM)
  Compute CoM Trajectory/1(CoM pos) -> Compute Output State/1(pos_CoM)
  Compute CoM Trajectory/2(CoM traj) -> trajCom_des/1
  Compute Output State/5(J) -> Delay1/1
  Link State Bus Deserialize/1 -> State-Machine/6(linkPose)
  link_state_other/1 -> Link State Bus Deserialize1/1
  Link State Bus Deserialize1/1 -> State-Machine/7(linkPoseDes)
  Delay/1 -> Link State Bus Deserialize/1
  Delay1/1 -> State-Machine/5(J)
  State-Machine/9(H) -> QP/1
  State-Machine/10(f) -> QP/2
  State-Machine/11(Aineq) -> QP/3
  State-Machine/12(bineq) -> QP/4
  State-Machine/7(phiOut) -> MatchSignalSizes/1, sum/1
  State-Machine/6(Deltat) -> Product/1
  Product/1 -> sum/2
  State-Machine/13(jointPose_des_old) -> sum1/1
  sum/1 -> Switch2/1, Product1/2
  Product1/1 -> sum1/2
  State-Machine/14(jointPose_delta) -> Product1/1
  State-Machine/1(jointPos_des) -> Switch1/3, Compute CoM Trajectory/1(Joint configuration), Compute Output State/2(jointPos)
  State-Machine/15(useQP) -> Switch2/2, Switch1/2
  sum1/1 -> Switch1/1
  Delay2/1 -> State-Machine/9(phiOld)
  Constant/1 -> Delay2/2
  QP/1 -> MatchSignalSizes/2
  MatchSignalSizes/1 -> Product/2
  State Bus Deserializer/1 -> State-Machine/2(w_H_base)
  State-Machine/8(phiNotQP) -> Delay2/1, phi/1, Switch2/3
  Link State Bus Deserialize1/2 -> State-Machine/8(linkVelocityDes)

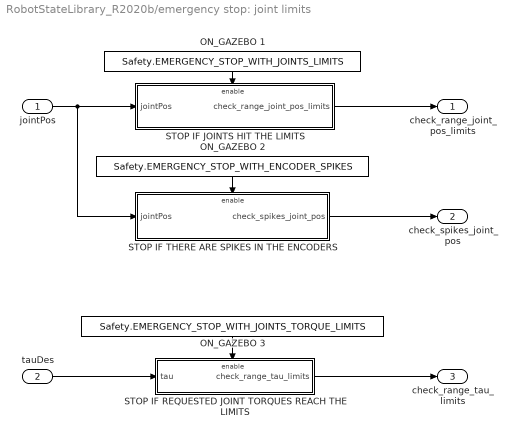
== system RobotStateLibrary_R2020b/emergency stop: joint limits ==
  jointPos : Inport
  tauDes : Inport  Port=2
  ON_GAZEBO 1 : Constant  Value=Safety.EMERGENCY_STOP_WITH_JOINTS_LIMITS
  ON_GAZEBO 2 : Constant  Value=Safety.EMERGENCY_STOP_WITH_ENCODER_SPIKES
  ON_GAZEBO 3 : Constant  Value=Safety.EMERGENCY_STOP_WITH_JOINTS_TORQUE_LIMITS
  STOP IF JOINTS HIT THE LIMITS : Subsystem
  STOP IF REQUESTED JOINT TORQUES REACH THE LIMITS : Subsystem
  STOP IF THERE ARE SPIKES IN THE ENCODERS : Subsystem
  check_range_joint_pos_limits : Outport
  check_spikes_joint_pos : Outport  Port=2
  check_range_tau_limits : Outport  Port=3
  wires:
  ON_GAZEBO 1/1 -> STOP IF JOINTS HIT THE LIMITS/Enable
  jointPos/1 -> STOP IF THERE ARE SPIKES IN THE ENCODERS/1(jointPos), STOP IF JOINTS HIT THE LIMITS/1(jointPos)
  ON_GAZEBO 2/1 -> STOP IF THERE ARE SPIKES IN THE ENCODERS/Enable
  ON_GAZEBO 3/1 -> STOP IF REQUESTED JOINT TORQUES REACH THE LIMITS/Enable
  tauDes/1 -> STOP IF REQUESTED JOINT TORQUES REACH THE LIMITS/1(tau)
  STOP IF JOINTS HIT THE LIMITS/1(check_range_joint_pos_limits) -> check_range_joint_pos_limits/1
  STOP IF THERE ARE SPIKES IN THE ENCODERS/1(check_spikes_joint_pos) -> check_spikes_joint_pos/1
  STOP IF REQUESTED JOINT TORQUES REACH THE LIMITS/1(check_range_tau_limits) -> check_range_tau_limits/1

== system RobotStateLibrary_R2020b/Compute State Velocity/Contacts Jacobians ==
  jointPos : Inport
  w_H_b : Inport  Port=2
  Jacobian Contact 1 : WBToolboxLibrary/Model/Jacobians/Jacobian  frameName=frameName1
      settings: SourceProductName=WholeBodyToolbox
  Jacobian Contact 2 : WBToolboxLibrary/Model/Jacobians/Jacobian  frameName=frameName2
      settings: SourceProductName=WholeBodyToolbox
  J_contact_1 : Outport  VectorParamsAs1DForOutWhenUnconnected=off
  J_contact_2 : Outport  Port=2  VectorParamsAs1DForOutWhenUnconnected=off
  wires:
  Jacobian Contact 1/1 -> J_contact_1/1
  Jacobian Contact 2/1 -> J_contact_2/1
  w_H_b/1 -> Jacobian Contact 2/1, Jacobian Contact 1/1
  jointPos/1 -> Jacobian Contact 1/2, Jacobian Contact 2/2

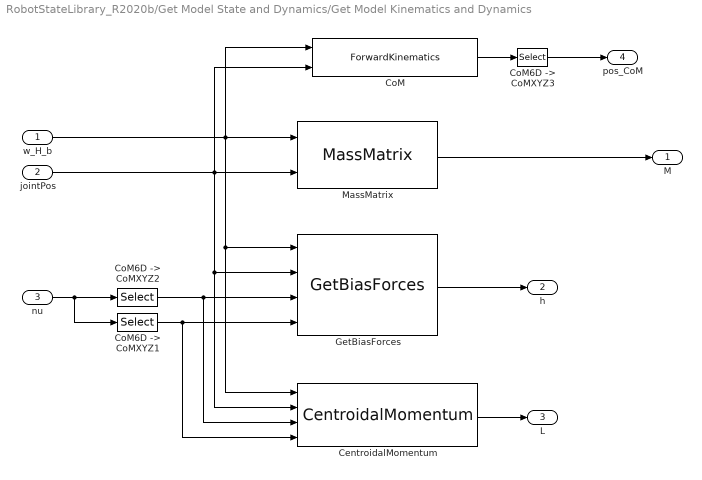
== system RobotStateLibrary_R2020b/Get Model State and Dynamics/Get Model Kinematics and Dynamics ==
  w_H_b : Inport
  jointPos : Inport  Port=2
  nu : Inport  Port=3
  CentroidalMomentum : WBToolboxLibrary/Model/Dynamics/CentroidalMomentum
      settings: SourceProductName=WholeBodyToolbox
  CoM : WBToolboxLibrary/Model/Kinematics/ForwardKinematics  frameName='com'
      settings: SourceProductName=WholeBodyToolbox
  "CoM6D -> CoMXYZ1" : Selector  IndexOptions=Starting index (dialog)  Indices=7  OutputSizes=1
  "CoM6D -> CoMXYZ2" : Selector  IndexOptions=Index vector (dialog)  Indices=[1 2 3 4 5 6]  OutputSizes=1
  "CoM6D -> CoMXYZ3" : Selector  NumberOfDimensions=2  InputPortWidth=7  IndexOptions=Index vector (dialog),Index vector (dialog)  Indices=[1 2 3],[4]  OutputSizes=1,1
  GetBiasForces : WBToolboxLibrary/Model/Dynamics/GetBiasForces
      settings: SourceProductName=WholeBodyToolbox
  MassMatrix : WBToolboxLibrary/Model/Dynamics/MassMatrix
      settings: SourceProductName=WholeBodyToolbox
  M : Outport  VectorParamsAs1DForOutWhenUnconnected=off
  h : Outport  Port=2  VectorParamsAs1DForOutWhenUnconnected=off
  L : Outport  Port=3  VectorParamsAs1DForOutWhenUnconnected=off
  pos_CoM : Outport  Port=4  VectorParamsAs1DForOutWhenUnconnected=off
  wires:
  CentroidalMomentum/1 -> L/1
  GetBiasForces/1 -> h/1
  w_H_b/1 -> CoM/1, CentroidalMomentum/1, GetBiasForces/1, MassMatrix/1
  jointPos/1 -> CoM/2, CentroidalMomentum/2, GetBiasForces/2, MassMatrix/2
  "CoM6D -> CoMXYZ2"/1 -> CentroidalMomentum/3, GetBiasForces/3
  "CoM6D -> CoMXYZ1"/1 -> CentroidalMomentum/4, GetBiasForces/4
  nu/1 -> "CoM6D -> CoMXYZ1"/1, "CoM6D -> CoMXYZ2"/1
  MassMatrix/1 -> M/1
  CoM/1 -> "CoM6D -> CoMXYZ3"/1
  "CoM6D -> CoMXYZ3"/1 -> pos_CoM/1

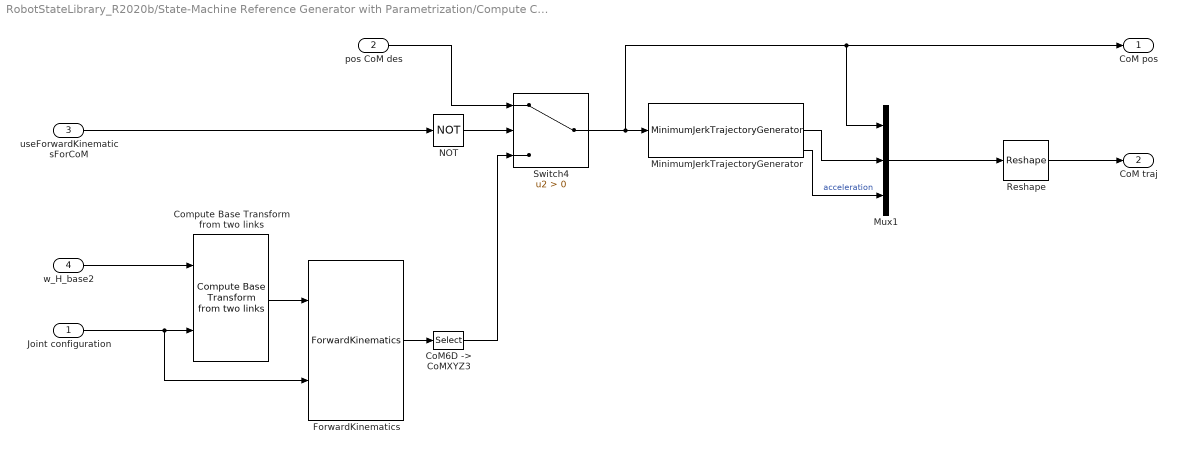
== system RobotStateLibrary_R2020b/State-Machine Reference Generator with Parametrization/Compute CoM Trajectory ==
  Joint configuration : Inport
  pos CoM des : Inport  Port=2
  useForwardKinematicsForCoM : Inport  Port=3
  w_H_base2 : Inport  Port=4
  "CoM6D -> CoMXYZ3" : Selector  NumberOfDimensions=2  InputPortWidth=7  IndexOptions=Index vector (dialog),Index vector (dialog)  Indices=[1 2 3],[4]  OutputSizes=1,1
  Compute Base Transform from two links : $bdroot/Compute Base Transform from two links  frameName1=frameName1  frameName2=frameName2
  ForwardKinematics : WBToolboxLibrary/Model/Kinematics/ForwardKinematics  frameName='com'
      settings: SourceProductName=WholeBodyToolbox
  MinimumJerkTrajectoryGenerator : WBToolboxLibrary/Utilities/MinimumJerkTrajectoryGenerator  externalSettlingTime=off  settlingTime=settlingTime  sampleTime=sampleTime  resetOnSettlingTime=off  firstDerivatives=on  secondDerivatives=on  explicitInitialValue=off
      settings: SourceProductName=WholeBodyToolbox
  Mux1 : Mux  Inputs=3
  NOT : Logic  Operator=NOT  IconShape=distinctive  AllPortsSameDT=off  OutDataTypeStr=boolean
  Reshape : Reshape  OutputDimensionality=Customize  OutputDimensions=[3,3]
  Switch4 : Switch  Criteria=u2 > Threshold
  CoM pos : Outport
  CoM traj : Outport  Port=2
  wires:
  Compute Base Transform from two links/1 -> ForwardKinematics/1
  Reshape/1 -> CoM traj/1
  Joint configuration/1 -> Compute Base Transform from two links/2, ForwardKinematics/2
  "CoM6D -> CoMXYZ3"/1 -> Switch4/3
  w_H_base2/1 -> Compute Base Transform from two links/1
  Mux1/1 -> Reshape/1
  pos CoM des/1 -> Switch4/1
  NOT/1 -> Switch4/2
  ForwardKinematics/1 -> "CoM6D -> CoMXYZ3"/1
  useForwardKinematicsForCoM/1 -> NOT/1
  MinimumJerkTrajectoryGenerator/2 -> Mux1/2
  MinimumJerkTrajectoryGenerator/3 -> Mux1/3  "acceleration"
  Switch4/1 -> Mux1/1, CoM pos/1, MinimumJerkTrajectoryGenerator/1

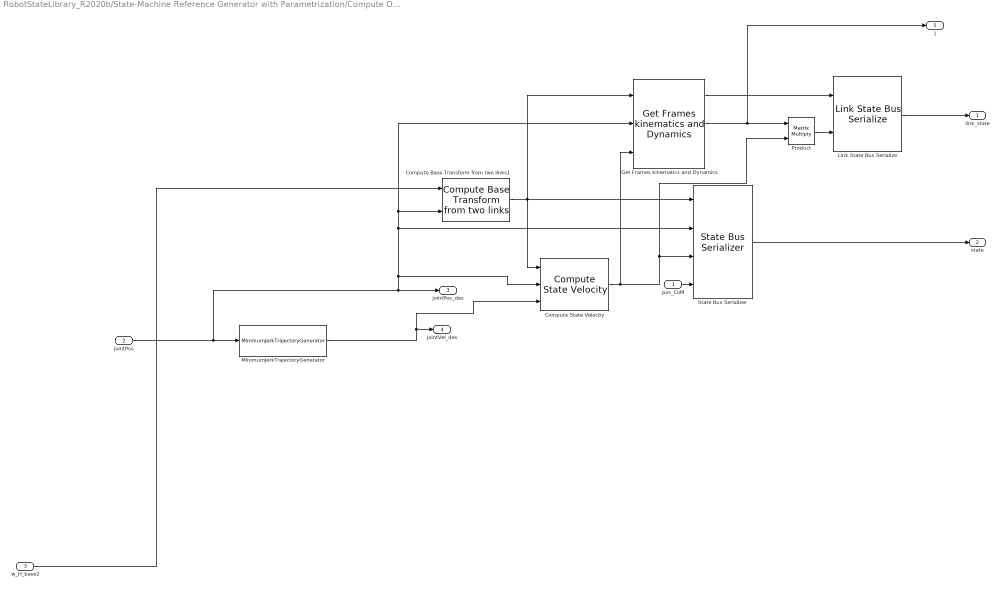
== system RobotStateLibrary_R2020b/State-Machine Reference Generator with Parametrization/Compute Output State ==
  pos_CoM : Inport
  jointPos : Inport  Port=2
  w_H_base2 : Inport  Port=3
  Compute Base Transform from two links1 : $bdroot/Compute Base Transform from two links  frameName1=frameName1  frameName2=frameName2
  Compute State Velocity : $bdroot/Compute State Velocity  frameName1=frameName1  frameName2=frameName2  regularization=regularization
  Get Frames kinematics and Dynamics : $bdroot/Get Frames kinematics and Dynamics  frame1=frame1  frame2=frame2  frame3=frame3  frame4=frame4  nDoF=ROBOT_DOF
  Link State Bus Serialize : $bdroot/Link State Bus Serialize  SystemSampleTime=-1  VariantActivationTime=update diagram  Latency=0  AutoFrameSizeCalculation=off
  MinimumJerkTrajectoryGenerator : WBToolboxLibrary/Utilities/MinimumJerkTrajectoryGenerator  externalSettlingTime=off  settlingTime=settlingTime  sampleTime=sampleTime  resetOnSettlingTime=off  firstDerivatives=on  secondDerivatives=on  explicitInitialValue=off
      settings: SourceProductName=WholeBodyToolbox
  Product : Product  Multiplication=Matrix(*)
  State Bus Serializer : $bdroot/State Bus Serializer  SystemSampleTime=-1  VariantActivationTime=update diagram  Latency=0  AutoFrameSizeCalculation=off
  link_state : Outport
  state : Outport  Port=2
  jointPos_des : Outport  Port=3
  jointVel_des : Outport  Port=4
  J : Outport  Port=5
  wires:
  Product/1 -> Link State Bus Serialize/2
  Compute Base Transform from two links1/1 -> Compute State Velocity/1, State Bus Serializer/1, Get Frames kinematics and Dynamics/1
  w_H_base2/1 -> Compute Base Transform from two links1/1
  Get Frames kinematics and Dynamics/1 -> Link State Bus Serialize/1
  pos_CoM/1 -> State Bus Serializer/4
  Link State Bus Serialize/1 -> link_state/1
  State Bus Serializer/1 -> state/1
  MinimumJerkTrajectoryGenerator/2 -> jointVel_des/1, Compute State Velocity/3
  Get Frames kinematics and Dynamics/2 -> J/1, Product/1
  Compute State Velocity/1 -> State Bus Serializer/3, Product/2, Get Frames kinematics and Dynamics/3
  jointPos/1 -> State Bus Serializer/2, Get Frames kinematics and Dynamics/2, Compute Base Transform from two links1/2, Compute State Velocity/2, jointPos_des/1, MinimumJerkTrajectoryGenerator/1

== system RobotStateLibrary_R2020b/emergency stop: joint limits/STOP IF JOINTS HIT THE LIMITS ==
  jointPos : Inport
  Enable : EnablePort
  Assertion : Assertion
  GetLimits : WBToolboxLibrary/States/GetLimits  limitsSource=ControlBoard  limitsType=Position
      settings: SourceProductName=WholeBodyToolbox
  MATLAB Function : MATLAB Function  TreatAsAtomicUnit=on
  Unit Delay : UnitDelay  InitialCondition=1  SampleTime=Config.tStep  HasFrameUpgradeWarning=on
  index1 : Constant  Value=Safety.jointLimitTollerance  VectorParams1D=off
  check_range_joint_pos_limits : Outport
  wires:
  jointPos/1 -> MATLAB Function/3(u)
  MATLAB Function/1(inRange) -> Unit Delay/1
  index1/1 -> MATLAB Function/4(tol)
  MATLAB Function/2(res_check_range) -> check_range_joint_pos_limits/1
  Unit Delay/1 -> Assertion/1
  GetLimits/1 -> MATLAB Function/1(umin)
  GetLimits/2 -> MATLAB Function/2(umax)

== system RobotStateLibrary_R2020b/emergency stop: joint limits/STOP IF REQUESTED JOINT TORQUES REACH THE LIMITS ==
  tau : Inport
  Enable : EnablePort
  Assertion : Assertion
  MATLAB Function : MATLAB Function  TreatAsAtomicUnit=on
  ON_GAZEBO 1 : Constant  Value=Safety.torqueSaturation
  ON_GAZEBO 3 : Constant  Value=-Safety.torqueSaturation
  Unit Delay : UnitDelay  InitialCondition=1  SampleTime=Config.tStep  HasFrameUpgradeWarning=on
  index1 : Constant  Value=ConfigRobot1.Safety.jointTorqueLimitTollerance  VectorParams1D=off
  check_range_tau_limits : Outport
  wires:
  tau/1 -> MATLAB Function/3(u)
  MATLAB Function/1(inRange) -> Unit Delay/1
  index1/1 -> MATLAB Function/4(tol)
  MATLAB Function/2(res_check_range) -> check_range_tau_limits/1
  Unit Delay/1 -> Assertion/1
  ON_GAZEBO 3/1 -> MATLAB Function/1(umin)
  ON_GAZEBO 1/1 -> MATLAB Function/2(umax)
